simulink model "ModellVergleich2"  (Simulink 9.3)
settings: Solver=ode45  StartTime=0.0  StopTime=10.0  MaxStep=1e-3  RelTol=1e-3
values from neighbouring files (symbols this model uses):
  B_1 = 2.39e6    (= 2390000)    [A2Main.m]
  C_o = 36.5e6    (= 36500000)    [A2Main.m]
  C_p = 75e6    (= 75000000)    [A2Main.m]
  h_matrix = inv(A) * (phi_matrix - eye(size(phi_matrix,1))) * B    [A2Main.m]
  M_g = M_k + M_p    (= 268.7)    [A2Main.m]
  phi_matrix = expm(A * T_a)    [A2Main.m]
  T_a = 0.015    [A2Main.m]
  U_step = 5e-4    (= 0.0005)    [A2Main.m]
undefined symbols (not defined in the file or in its folder): C, D
settings Model: Creator=wredi  LastModifiedBy=wredi
settings DataIOCC: SaveFormat=Dataset  SignalLoggingSaveFormat=Dataset  ReturnWorkspaceOutputs=on
settings DebuggingCC: UnderspecifiedInitializationDetection=Simplified  MergeDetectMultiDrivingBlocksExec=error  FcnCallInpInsideContextMsg=error  SFUnexpectedBacktrackingDiag=error  SFNoUnconditionalDefaultTransitionDiag=error  SFExecutionAtInitializationDiag=warning
settings HardwareCC: ProdBitPerPointer=64  ProdBitPerSizeT=64  ProdBitPerPtrDiffT=64  ProdLargestAtomicFloat=Float  ProdIntDivRoundTo=Zero  ProdEndianess=LittleEndian  ProdWordSize=64  ProdHWDeviceType=Intel->x86-64 (Windows64)
settings ModelReferenceCC: PropagateSignalLabelsOutOfModel=on
settings SFSimCC: SimUseLocalCustomCode=on
settings RTWCC: RTWUseLocalCustomCode=on
settings CodeAppCC: StateflowObjectComments=off
settings GRTTargetCC: TargetLangStandard=C99 (ISO)  CombineOutputUpdateFcns=on  GRTInterface=off
settings ConfigComp: CovMetricSettings=dwe  CovHtmlReporting=off  CovSaveCumulativeToWorkspaceVar=off  CovSaveSingleToWorkspaceVar=off  CovExternalEMLEnable=on

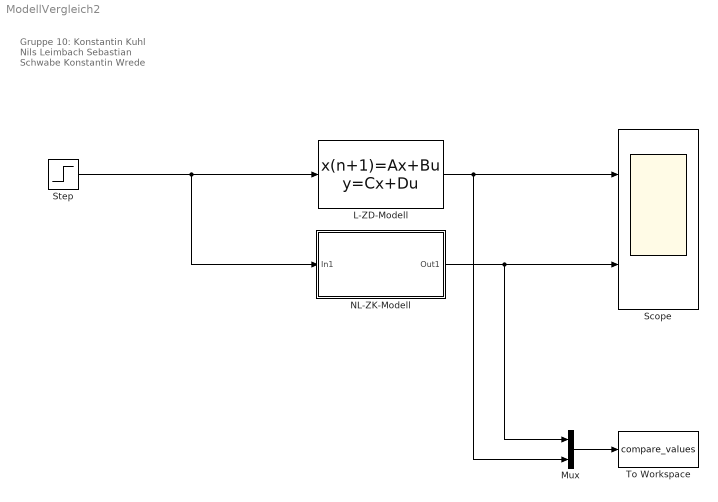
== system ModellVergleich2 ==
  note: Gruppe 10:
      | Konstantin Kuhl
      | Nils Leimbach
      | Sebastian Schwabe
      | Konstantin Wrede
  L-ZD-Modell : DiscreteStateSpace  A=phi_matrix  B=h_matrix  C=C  D=D  SampleTime=T_a
  Mux : Mux  Inputs=2
  "NL-ZK-Modell " : Subsystem
  Scope : Scope  NumInputPorts=2
  Step : Step  After=U_step  SampleTime=0
  To Workspace : ToWorkspace  VariableName=compare_values  SaveFormat=Structure With Time  SampleTime=-1
  wires:
  L-ZD-Modell/1 -> Mux/2, Scope/1
  "NL-ZK-Modell "/1(Out1) -> Mux/1, Scope/2
  Step/1 -> "NL-ZK-Modell "/1(In1), L-ZD-Modell/1
  Mux/1 -> To Workspace/1

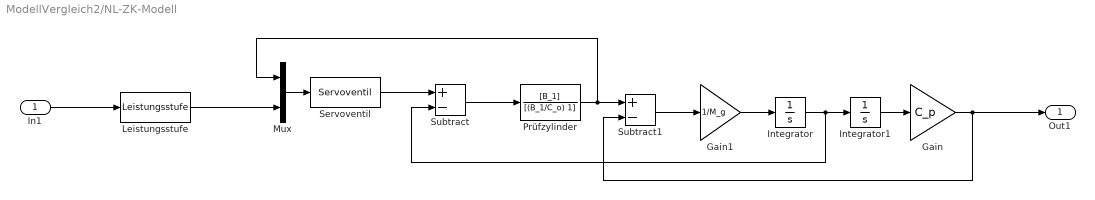
== system ModellVergleich2/NL-ZK-Modell  ==
  In1 : Inport
  Gain : Gain  Gain=C_p
  Gain1 : Gain  Gain=1/M_g
  Integrator : Integrator
  Integrator1 : Integrator
  Leistungsstufe : MATLABFcn  MATLABFcn=Leistungsstufe  OutputDimensions=1
  Mux : Mux  Inputs=2
  Prüfzylinder : TransferFcn  Numerator=[B_1]  Denominator=[(B_1/C_o) 1]
  "Servoventil " : MATLABFcn  MATLABFcn=Servoventil  OutputDimensions=1  Output1D=off
  Subtract : Sum  Inputs=+-
  Subtract1 : Sum  Inputs=+-
  Out1 : Outport
  wires:
  Subtract/1 -> Prüfzylinder/1
  Integrator/1 -> Subtract/2, Integrator1/1
  Subtract1/1 -> Gain1/1
  Integrator1/1 -> Gain/1
  Gain1/1 -> Integrator/1
  Prüfzylinder/1 -> Mux/1, Subtract1/1
  Leistungsstufe/1 -> Mux/2
  Gain/1 -> Out1/1, Subtract1/2
  "Servoventil "/1 -> Subtract/1
  Mux/1 -> "Servoventil "/1
  In1/1 -> Leistungsstufe/1
